simulink model "model1"  (R2022a)
settings: Solver=VariableStepAuto  StartTime=0.0  StopTime=0.3  RelTol=1e-3
values from neighbouring files (symbols this model uses):
  T = 0.005    [config.m]
  W = tf(b, a, T)    [config.m]
  W_1 = K_1/(Tau_1*s + 1)    [config.m]
  W_2 = K_2/(Tau_2*s + 1)    [config.m]
  W_3 = K_3/s    [config.m]
settings Model: Creator=Vvlad  LastModifiedBy=Vvlad

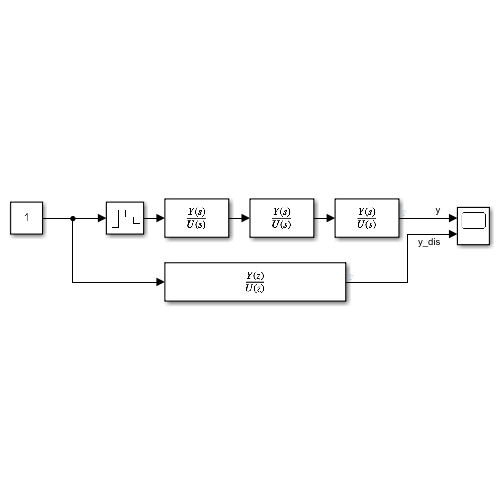
[thumbnail: Simulink's stored preview of the top-level diagram]
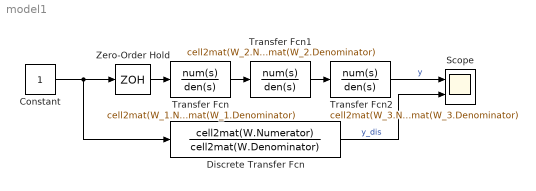
== system model1 ==
  Constant : Constant
  Discrete Transfer Fcn : DiscreteTransferFcn  Numerator=cell2mat(W.Numerator)  Denominator=cell2mat(W.Denominator)  SampleTime=T
  Scope : Scope  NumInputPorts=2
  Transfer Fcn : TransferFcn  Numerator=cell2mat(W_1.Numerator)  Denominator=cell2mat(W_1.Denominator)
  Transfer Fcn1 : TransferFcn  Numerator=cell2mat(W_2.Numerator)  Denominator=cell2mat(W_2.Denominator)
  Transfer Fcn2 : TransferFcn  Numerator=cell2mat(W_3.Numerator)  Denominator=cell2mat(W_3.Denominator)
  Zero-Order Hold : ZeroOrderHold  SampleTime=T
  wires:
  Constant/1 -> Discrete Transfer Fcn/1, Zero-Order Hold/1
  Zero-Order Hold/1 -> Transfer Fcn/1
  Transfer Fcn/1 -> Transfer Fcn1/1
  Transfer Fcn1/1 -> Transfer Fcn2/1
  Discrete Transfer Fcn/1 -> Scope/2  "y_dis"
  Transfer Fcn2/1 -> Scope/1  "y"
